simulink model "controller"  (Simulink 8.1)
settings: Solver=ode45  StartTime=0.0  StopTime=10.0  RelTol=1e-3
settings Model: Creator=eiseles  LastModifiedBy=eiseles
settings DataIOCC: SignalLoggingSaveFormat=Dataset
settings OptimizationCC: ExpressionDepthLimit=128
settings DebuggingCC: FcnCallInpInsideContextMsg=EnableAllAsError
settings GRTTargetCC: CombineOutputUpdateFcns=on  GRTInterface=off

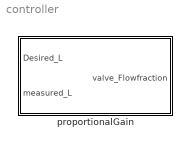
== system controller ==
  proportionalGain : Subsystem

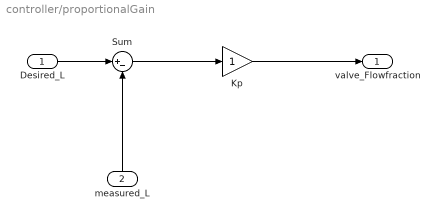
== system controller/proportionalGain ==
  Desired_L : Inport
  measured_L : Inport  Port=2
  Kp : Gain
  Sum : Sum  Inputs=|+-
  valve_Flowfraction : Outport
  wires:
  Sum/1 -> Kp/1
  measured_L/1 -> Sum/2
  Desired_L/1 -> Sum/1
  Kp/1 -> valve_Flowfraction/1
